simulink model "APP_MyApplication"  (R2018b)
settings: Solver=VariableStepDiscrete  StartTime=0.0  StopTime=10  RelTol=1e-3
PreLoadFcn:
  | if(exist('MBDS_ModelCallback', 'file')), MBDS_ModelCallback('PreLoad'); end;
PostLoadFcn:
  | if(exist('MBDS_ModelCallback', 'file')), MBDS_ModelCallback('PostLoad'); end;
InitFcn:
  | if(exist('MBDS_ModelCallback', 'file')), MBDS_ModelCallback('Init'); end;
StartFcn:
  | if(exist('MBDS_ModelCallback', 'file')), MBDS_ModelCallback('Start'); end;
StopFcn:
  | if(exist('MBDS_ModelCallback', 'file')), MBDS_ModelCallback('Stop'); end;
undefined symbols (not defined in the file): sigbuilder_block, Ts
libraries: KIBES_Signal x499, simulink x8
(part 2 of 10)

== system APP_MyApplication/Model/APP_MyApplication_/D-CAN(1) ==
  note: 18 01 01 F1
  Add : Sum  InitFcn=|  OutDataTypeStr=Inherit: Inherit via back propagation  SaturateOnIntegerOverflow=on
      | if(exist('MBDS_BlockCallback', 'file'))
      |    MBDS_BlockCallback('Update', gcb);  
      | end
      settings: AttributesFormatString=Saturate: %<SaturateOnIntegerOverflow>
  Constant1 : Constant  InitFcn=|  Value=0  OutDataTypeStr=boolean
      | if(exist('MBDS_BlockCallback', 'file'))
      |    MBDS_BlockCallback('Update', gcb);  
      | end
  Constant2 : Constant  InitFcn=|  OutDataTypeStr=boolean
      | if(exist('MBDS_BlockCallback', 'file'))
      |    MBDS_BlockCallback('Update', gcb);  
      | end
  Constant3 : Constant  InitFcn=|  Value=2  OutDataTypeStr=uint8
      | if(exist('MBDS_BlockCallback', 'file'))
      |    MBDS_BlockCallback('Update', gcb);  
      | end
  Constant4 : Constant  InitFcn=|  Value=3  OutDataTypeStr=uint8
      | if(exist('MBDS_BlockCallback', 'file'))
      |    MBDS_BlockCallback('Update', gcb);  
      | end
  Constant5 : Constant  InitFcn=|  Value=4  OutDataTypeStr=uint8
      | if(exist('MBDS_BlockCallback', 'file'))
      |    MBDS_BlockCallback('Update', gcb);  
      | end
  Constant6 : Constant  InitFcn=|  Value=1234  OutDataTypeStr=uint32
      | if(exist('MBDS_BlockCallback', 'file'))
      |    MBDS_BlockCallback('Update', gcb);  
      | end
  Constant7 : Constant  InitFcn=|  OutDataTypeStr=boolean
      | if(exist('MBDS_BlockCallback', 'file'))
      |    MBDS_BlockCallback('Update', gcb);  
      | end
  Constant9 : Constant  InitFcn=|  OutDataTypeStr=uint32
      | if(exist('MBDS_BlockCallback', 'file'))
      |    MBDS_BlockCallback('Update', gcb);  
      | end
  Data Type Conversion : DataTypeConversion  InitFcn=|  SaturateOnIntegerOverflow=on
      | try
      |    MBDS_BlockCallback('Update', gcb);
      | end
      settings: AttributesFormatString=Saturate: %<SaturateOnIntegerOverflow>
  NOT : Subsystem  InitFcn=|  mask(NOT){MBDS_LibraryBlock=on, BitwiseMode=off, Inputs=1, UseBitMask=off, BitMask='A1', OutDataTypeStr=Inherit: Inherit via back propagation, MBDS_BlockVersion=07.21.05}
      | if(exist('MBDS_BlockCallback', 'file'))
      |    MBDS_BlockCallback('Update', gcb);
      | end
      mask prompts: MBDS_LibraryBlock "MBDS library block"; BitwiseMode "Use 'bitwise' mode"; Inputs "Number of input ports:"; UseBitMask "Use bit mask"; BitMask "Bit mask:"; OutDataTypeStr "Output data type:"; MBDS_BlockVersion "Version:"
      mask help: Logical or bitwise NOT operator. The input value is inverted. In bitwise mode all bits of the input signal are inverted.
      mask init: same as APP_MyApplication/Model/APP_MyApplication_/OR
      mask Help: eval(['open([workdir(''library_dir:''),''\Blockset\help\'',get_param(gcb,''MaskType''),''.html''])'])
      mask Callback BitwiseMode:
      | if(exist('MBDS_BlockCallback', 'file'))
      |    MBDS_BlockCallback('BitwiseMode', gcb);
      | end
      mask TypeOptions OutDataTypeStr: Inherit: Inherit via back propagation | int8 | uint8 | int16 | uint16 | int32 | uint32 | boolean
      mask Callback OutDataTypeStr:
      | % Adopt Value
      | if(exist('MBDS_BlockCallback', 'file'))
      |    MBDS_BlockCallback('OutDataTypeStr', gcb);
      | end
      mask DialogControl ParameterTabVar0 Prompt: Main
      mask DialogControl ParameterTabVar01 Prompt: Signal Attributes
      mask DialogControl ParameterTabVar012 Prompt: Version
      mask Display:
      | % Show icon or block text
      | disp('NOT')
  in_DCAN.TX_Gen.DGenTx_4.MessageState : KIBES_Signal/KIBES_Signal  MBDS_LibraryBlock=on  DatabaseKey=271  SignalName=DCAN.TX_Gen.DGenTx_4.MessageState  SymbolName=DCAN_TX_Gen_DGenTx_4_MessageState_000271  DataType=uint16  Init=0  Slope=1  Bias=0  DataSize=1  fpDataType=uint16  BlockIOType=Inport  DeviceType=0
  in_DCAN.TX_Gen.DGenTx_4.Val1 : KIBES_Signal/KIBES_Signal  MBDS_LibraryBlock=on  DatabaseKey=272  SignalName=DCAN.TX_Gen.DGenTx_4.Val1  SymbolName=DCAN_TX_Gen_DGenTx_4_Val1_000272  DataType=uint32  Init=0  Slope=1  Bias=0  DataSize=1  fpDataType=uint32  BlockIOType=Inport  DeviceType=0
  in_IN_DCAN.RX_Gen.Test1.MessageState : KIBES_Signal/KIBES_Signal  MBDS_LibraryBlock=on  DatabaseKey=10  SignalName=IN_DCAN.RX_Gen.Test1.MessageState  SymbolName=IN_DCAN_RX_Gen_Test1_MessageState_000010  DataType=uint16  Init=0  Slope=1  Bias=0  DataSize=1  fpDataType=uint16  BlockIOType=Inport  DeviceType=0
  in_IN_DCAN.RX_Gen.Test1.Val1 : KIBES_Signal/KIBES_Signal  MBDS_LibraryBlock=on  DatabaseKey=11  SignalName=IN_DCAN.RX_Gen.Test1.Val1  SymbolName=IN_DCAN_RX_Gen_Test1_Val1_000011  DataType=uint8  Init=0  Slope=1  Bias=0  DataSize=1  fpDataType=uint8  BlockIOType=Inport  DeviceType=0
  in_IN_DCAN.TX_Gen.GenericTxMessage.MessageState : KIBES_Signal/KIBES_Signal  MBDS_LibraryBlock=on  DatabaseKey=3  SignalName=IN_DCAN.TX_Gen.GenericTxMessage.MessageState  SymbolName=IN_DCAN_TX_Gen_GenericTxMessage_MessageState_000003  DataType=uint16  Init=0  Slope=1  Bias=0  DataSize=1  fpDataType=uint16  BlockIOType=Inport  DeviceType=0
  in_STIMD.GenTxCycleTime : KIBES_Signal/KIBES_Signal  MBDS_LibraryBlock=on  DatabaseKey=576  SignalName=STIMD.GenTxCycleTime  SymbolName=STIMD_GenTxCycleTime_000576  DataType=uint16  Init=100  Slope=1  Bias=0  DataSize=1  fpDataType=uint16  BlockIOType=Inport  DeviceType=2
  out_DCAN.TX_Gen.DGenTx_4.MessageEnable : KIBES_Signal/KIBES_Signal  MBDS_LibraryBlock=on  DatabaseKey=270  SignalName=DCAN.TX_Gen.DGenTx_4.MessageEnable  SymbolName=DCAN_TX_Gen_DGenTx_4_MessageEnable_000270  DataType=boolean  Init=0  Slope=1  Bias=0  DataSize=1  fpDataType=boolean  BlockIOType=Outport  DeviceType=0
  out_DCAN.TX_Gen.DGenTx_4.Val1 : KIBES_Signal/KIBES_Signal  MBDS_LibraryBlock=on  DatabaseKey=272  SignalName=DCAN.TX_Gen.DGenTx_4.Val1  SymbolName=DCAN_TX_Gen_DGenTx_4_Val1_000272  DataType=uint32  Init=0  Slope=1  Bias=0  DataSize=1  fpDataType=uint32  BlockIOType=Outport  DeviceType=0
  out_DCAN.TX_Gen.GenericTxMessage.CycleTime : KIBES_Signal/KIBES_Signal  MBDS_LibraryBlock=on  DatabaseKey=575  SignalName=DCAN.TX_Gen.GenericTxMessage.CycleTime  SymbolName=DCAN_TX_Gen_GenericTxMessage_CycleTime_000575  DataType=uint16  Init=0  Slope=1  Bias=0  DataSize=1  fpDataType=uint16  BlockIOType=Outport  DeviceType=0
  out_OUT_DCAN.RX_Gen.Test1.MessageEnable : KIBES_Signal/KIBES_Signal  MBDS_LibraryBlock=on  DatabaseKey=9  SignalName=OUT_DCAN.RX_Gen.Test1.MessageEnable  SymbolName=OUT_DCAN_RX_Gen_Test1_MessageEnable_000009  DataType=boolean  Init=0  Slope=1  Bias=0  DataSize=1  fpDataType=boolean  BlockIOType=Outport  DeviceType=0
  out_OUT_DCAN.TX_Gen.GenericTxMessage.MessageEnable : KIBES_Signal/KIBES_Signal  MBDS_LibraryBlock=on  DatabaseKey=2  SignalName=OUT_DCAN.TX_Gen.GenericTxMessage.MessageEnable  SymbolName=OUT_DCAN_TX_Gen_GenericTxMessage_MessageEnable_000002  DataType=boolean  Init=0  Slope=1  Bias=0  DataSize=1  fpDataType=boolean  BlockIOType=Outport  DeviceType=0
  out_OUT_DCAN.TX_Gen.GenericTxMessage.Val1 : KIBES_Signal/KIBES_Signal  MBDS_LibraryBlock=on  DatabaseKey=4  SignalName=OUT_DCAN.TX_Gen.GenericTxMessage.Val1  SymbolName=OUT_DCAN_TX_Gen_GenericTxMessage_Val1_000004  DataType=uint8  Init=0  Slope=1  Bias=0  DataSize=1  fpDataType=uint8  BlockIOType=Outport  DeviceType=0
  out_OUT_DCAN.TX_Gen.GenericTxMessage.Val2 : KIBES_Signal/KIBES_Signal  MBDS_LibraryBlock=on  DatabaseKey=5  SignalName=OUT_DCAN.TX_Gen.GenericTxMessage.Val2  SymbolName=OUT_DCAN_TX_Gen_GenericTxMessage_Val2_000005  DataType=uint8  Init=0  Slope=1  Bias=0  DataSize=1  fpDataType=uint8  BlockIOType=Outport  DeviceType=0
  out_OUT_DCAN.TX_Gen.GenericTxMessage.Val3 : KIBES_Signal/KIBES_Signal  MBDS_LibraryBlock=on  DatabaseKey=6  SignalName=OUT_DCAN.TX_Gen.GenericTxMessage.Val3  SymbolName=OUT_DCAN_TX_Gen_GenericTxMessage_Val3_000006  DataType=uint8  Init=0  Slope=1  Bias=0  DataSize=1  fpDataType=uint8  BlockIOType=Outport  DeviceType=0
  out_OUT_DCAN.TX_Gen.GenericTxMessage.Val4 : KIBES_Signal/KIBES_Signal  MBDS_LibraryBlock=on  DatabaseKey=7  SignalName=OUT_DCAN.TX_Gen.GenericTxMessage.Val4  SymbolName=OUT_DCAN_TX_Gen_GenericTxMessage_Val4_000007  DataType=uint8  Init=0  Slope=1  Bias=0  DataSize=1  fpDataType=uint8  BlockIOType=Outport  DeviceType=0
  out_OUT_DCAN.TX_Gen.GenericTxMessage.Val5 : KIBES_Signal/KIBES_Signal  MBDS_LibraryBlock=on  DatabaseKey=8  SignalName=OUT_DCAN.TX_Gen.GenericTxMessage.Val5  SymbolName=OUT_DCAN_TX_Gen_GenericTxMessage_Val5_000008  DataType=uint32  Init=0  Slope=1  Bias=0  DataSize=1  fpDataType=uint32  BlockIOType=Outport  DeviceType=0
  wires:
  Add/1 -> out_DCAN.TX_Gen.DGenTx_4.Val1/1
  in_DCAN.TX_Gen.DGenTx_4.Val1/1 -> Add/1
  Constant9/1 -> Add/2
  Constant6/1 -> out_OUT_DCAN.TX_Gen.GenericTxMessage.Val5/1
  in_STIMD.GenTxCycleTime/1 -> out_DCAN.TX_Gen.GenericTxMessage.CycleTime/1
  Data Type Conversion/1 -> NOT/1(u1)
  Constant5/1 -> out_OUT_DCAN.TX_Gen.GenericTxMessage.Val4/1
  Constant3/1 -> out_OUT_DCAN.TX_Gen.GenericTxMessage.Val2/1
  Constant7/1 -> out_OUT_DCAN.RX_Gen.Test1.MessageEnable/1
  in_IN_DCAN.RX_Gen.Test1.MessageState/1 -> Data Type Conversion/1
  Constant4/1 -> out_OUT_DCAN.TX_Gen.GenericTxMessage.Val3/1
  in_IN_DCAN.RX_Gen.Test1.Val1/1 -> out_OUT_DCAN.TX_Gen.GenericTxMessage.Val1/1
  NOT/1(y) -> out_OUT_DCAN.TX_Gen.GenericTxMessage.MessageEnable/1
  Constant2/1 -> out_DCAN.TX_Gen.DGenTx_4.MessageEnable/1

== system APP_MyApplication/Model/APP_MyApplication_/DM13 ==
  Constant1 : Constant  InitFcn=|  Value=0  OutDataTypeStr=boolean
      | if(exist('MBDS_BlockCallback', 'file'))
      |    MBDS_BlockCallback('Update', gcb);  
      | end
  Data Type Conversion : DataTypeConversion  InitFcn=|  SaturateOnIntegerOverflow=on
      | try
      |    MBDS_BlockCallback('Update', gcb);
      | end
      settings: AttributesFormatString=Saturate: %<SaturateOnIntegerOverflow>
  OR1 : Subsystem  InitFcn=|  mask(OR){MBDS_LibraryBlock=on, BitwiseMode=off, Inputs=2, UseBitMask=off, BitMask='A1', OutDataTypeStr=Inherit: Inherit via back propagation, MBDS_BlockVersion=07.21.05}
      | if(exist('MBDS_BlockCallback', 'file'))
      |    MBDS_BlockCallback('Update', gcb);
      | end
      mask prompts: MBDS_LibraryBlock "MBDS library block"; BitwiseMode "Use 'bitwise' mode"; Inputs "Number of input ports:"; UseBitMask "Use bit mask"; BitMask "Bit mask:"; OutDataTypeStr "Output data type:"; MBDS_BlockVersion "Version:"
      mask help: Logical or bitwise OR operator. For multiple inputs, operators are applied across the inputs. For a single input, operators are applied across the input vector. In bitwise mode a bit mask can be applied onto single input signals.
      mask init: same as APP_MyApplication/Model/APP_MyApplication_/OR
      mask Help: eval(['open([workdir(''library_dir:''),''\Blockset\help\'',get_param(gcb,''MaskType''),''.html''])'])
      mask Callback BitwiseMode:
      | if(exist('MBDS_BlockCallback', 'file'))
      |    MBDS_BlockCallback('BitwiseMode', gcb);
      | end
      mask Callback Inputs:
      | if(exist('MBDS_BlockCallback', 'file'))
      |    MBDS_BlockCallback('Inputs', gcb);
      | end
      mask Callback UseBitMask:
      | if(exist('MBDS_BlockCallback', 'file'))
      |    MBDS_BlockCallback('UseBitMask', gcb);
      | end
      mask Callback BitMask:
      | if(exist('MBDS_BlockCallback', 'file'))
      |    MBDS_BlockCallback('BitMask', gcb);
      | end
      mask TypeOptions OutDataTypeStr: Inherit: Inherit via back propagation | int8 | uint8 | int16 | uint16 | int32 | uint32 | boolean
      mask Callback OutDataTypeStr:
      | % Adopt Value
      | if(exist('MBDS_BlockCallback', 'file'))
      |    MBDS_BlockCallback('OutDataTypeStr', gcb);
      | end
      mask DialogControl ParameterTabVar0 Prompt: Main
      mask DialogControl ParameterTabVar01 Prompt: Signal Attributes
      mask DialogControl ParameterTabVar012 Prompt: Version
      mask Display:
      | % Show icon or block text
      | if(UseBitMask)
      |    if(isnumeric(BitMask))
      |       BitMaskString = ['0x',dec2hex(floor(BitMask))];
      |    elseif(ischar(BitMask))
      |       BitMaskString = ['0x',upper(BitMask)];
      |    else
      |       BitMaskString = '???';
      |    end
      |    disp(sprintf(['OR\n', BitMaskString]))
      | else
      |    disp('OR')
      | end
  in_DCAN.BusOffState : KIBES_Signal/KIBES_Signal  MBDS_LibraryBlock=on  DatabaseKey=639  SignalName=DCAN.BusOffState  SymbolName=DCAN_BusOffState_000639  DataType=boolean  Init=0  Slope=1  Bias=0  DataSize=1  fpDataType=boolean  BlockIOType=Inport  DeviceType=0
  in_DCAN.GenericDM13RXMessage.CurrentDataLink : KIBES_Signal/KIBES_Signal  MBDS_LibraryBlock=on  DatabaseKey=366  SignalName=DCAN.GenericDM13RXMessage.CurrentDataLink  SymbolName=DCAN_GenericDM13RXMessage_CurrentDataLink_000366  DataType=boolean  Init=0  Slope=1  Bias=0  DataSize=1  fpDataType=boolean  BlockIOType=Inport  DeviceType=0
  in_DCAN.GenericDM13RXMessage.CurrentDataLink_DIAG : KIBES_Signal/KIBES_Signal  MBDS_LibraryBlock=on  DatabaseKey=365  SignalName=DCAN.GenericDM13RXMessage.CurrentDataLink_DIAG  SymbolName=DCAN_GenericDM13RXMessage_CurrentDataLink_DIAG_000365  DataType=uint16  Init=1  Slope=1  Bias=0  DataSize=1  fpDataType=uint16  BlockIOType=Inport  DeviceType=0
  in_DCAN.GenericDM13RXMessage.DataChangeIndicator : KIBES_Signal/KIBES_Signal  MBDS_LibraryBlock=on  DatabaseKey=364  SignalName=DCAN.GenericDM13RXMessage.DataChangeIndicator  SymbolName=DCAN_GenericDM13RXMessage_DataChangeIndicator_000364  DataType=boolean  Init=0  Slope=1  Bias=0  DataSize=1  fpDataType=boolean  BlockIOType=Inport  DeviceType=0
  in_DCAN.GenericDM13RXMessage.DeviceState : KIBES_Signal/KIBES_Signal  MBDS_LibraryBlock=on  DatabaseKey=362  SignalName=DCAN.GenericDM13RXMessage.DeviceState  SymbolName=DCAN_GenericDM13RXMessage_DeviceState_000362  DataType=uint16  Init=0  Slope=1  Bias=0  DataSize=1  fpDataType=uint16  BlockIOType=Inport  DeviceType=0
  in_DCAN.GenericDM13RXMessage.ISO9141 : KIBES_Signal/KIBES_Signal  MBDS_LibraryBlock=on  DatabaseKey=361  SignalName=DCAN.GenericDM13RXMessage.ISO9141  SymbolName=DCAN_GenericDM13RXMessage_ISO9141_000361  DataType=boolean  Init=0  Slope=1  Bias=0  DataSize=1  fpDataType=boolean  BlockIOType=Inport  DeviceType=0
  in_DCAN.GenericDM13RXMessage.ISO9141_DIAG : KIBES_Signal/KIBES_Signal  MBDS_LibraryBlock=on  DatabaseKey=360  SignalName=DCAN.GenericDM13RXMessage.ISO9141_DIAG  SymbolName=DCAN_GenericDM13RXMessage_ISO9141_DIAG_000360  DataType=uint16  Init=1  Slope=1  Bias=0  DataSize=1  fpDataType=uint16  BlockIOType=Inport  DeviceType=0
  in_DCAN.GenericDM13RXMessage.J1587 : KIBES_Signal/KIBES_Signal  MBDS_LibraryBlock=on  DatabaseKey=359  SignalName=DCAN.GenericDM13RXMessage.J1587  SymbolName=DCAN_GenericDM13RXMessage_J1587_000359  DataType=boolean  Init=0  Slope=1  Bias=0  DataSize=1  fpDataType=boolean  BlockIOType=Inport  DeviceType=0
  in_DCAN.GenericDM13RXMessage.J1587_DIAG : KIBES_Signal/KIBES_Signal  MBDS_LibraryBlock=on  DatabaseKey=358  SignalName=DCAN.GenericDM13RXMessage.J1587_DIAG  SymbolName=DCAN_GenericDM13RXMessage_J1587_DIAG_000358  DataType=uint16  Init=1  Slope=1  Bias=0  DataSize=1  fpDataType=uint16  BlockIOType=Inport  DeviceType=0
  in_DCAN.GenericDM13RXMessage.J1850 : KIBES_Signal/KIBES_Signal  MBDS_LibraryBlock=on  DatabaseKey=357  SignalName=DCAN.GenericDM13RXMessage.J1850  SymbolName=DCAN_GenericDM13RXMessage_J1850_000357  DataType=boolean  Init=0  Slope=1  Bias=0  DataSize=1  fpDataType=boolean  BlockIOType=Inport  DeviceType=0
  in_DCAN.GenericDM13RXMessage.J1850_DIAG : KIBES_Signal/KIBES_Signal  MBDS_LibraryBlock=on  DatabaseKey=356  SignalName=DCAN.GenericDM13RXMessage.J1850_DIAG  SymbolName=DCAN_GenericDM13RXMessage_J1850_DIAG_000356  DataType=uint16  Init=1  Slope=1  Bias=0  DataSize=1  fpDataType=uint16  BlockIOType=Inport  DeviceType=0
  in_DCAN.GenericDM13RXMessage.J1922 : KIBES_Signal/KIBES_Signal  MBDS_LibraryBlock=on  DatabaseKey=355  SignalName=DCAN.GenericDM13RXMessage.J1922  SymbolName=DCAN_GenericDM13RXMessage_J1922_000355  DataType=boolean  Init=0  Slope=1  Bias=0  DataSize=1  fpDataType=boolean  BlockIOType=Inport  DeviceType=0
  in_DCAN.GenericDM13RXMessage.J1922_DIAG : KIBES_Signal/KIBES_Signal  MBDS_LibraryBlock=on  DatabaseKey=354  SignalName=DCAN.GenericDM13RXMessage.J1922_DIAG  SymbolName=DCAN_GenericDM13RXMessage_J1922_DIAG_000354  DataType=uint16  Init=1  Slope=1  Bias=0  DataSize=1  fpDataType=uint16  BlockIOType=Inport  DeviceType=0
  in_DCAN.GenericDM13RXMessage.Network1 : KIBES_Signal/KIBES_Signal  MBDS_LibraryBlock=on  DatabaseKey=353  SignalName=DCAN.GenericDM13RXMessage.Network1  SymbolName=DCAN_GenericDM13RXMessage_Network1_000353  DataType=boolean  Init=0  Slope=1  Bias=0  DataSize=1  fpDataType=boolean  BlockIOType=Inport  DeviceType=0
  in_DCAN.GenericDM13RXMessage.Network1_DIAG : KIBES_Signal/KIBES_Signal  MBDS_LibraryBlock=on  DatabaseKey=352  SignalName=DCAN.GenericDM13RXMessage.Network1_DIAG  SymbolName=DCAN_GenericDM13RXMessage_Network1_DIAG_000352  DataType=uint16  Init=1  Slope=1  Bias=0  DataSize=1  fpDataType=uint16  BlockIOType=Inport  DeviceType=0
  in_DCAN.GenericDM13RXMessage.Network2 : KIBES_Signal/KIBES_Signal  MBDS_LibraryBlock=on  DatabaseKey=351  SignalName=DCAN.GenericDM13RXMessage.Network2  SymbolName=DCAN_GenericDM13RXMessage_Network2_000351  DataType=boolean  Init=0  Slope=1  Bias=0  DataSize=1  fpDataType=boolean  BlockIOType=Inport  DeviceType=0
  in_DCAN.GenericDM13RXMessage.Network2_DIAG : KIBES_Signal/KIBES_Signal  MBDS_LibraryBlock=on  DatabaseKey=350  SignalName=DCAN.GenericDM13RXMessage.Network2_DIAG  SymbolName=DCAN_GenericDM13RXMessage_Network2_DIAG_000350  DataType=uint16  Init=1  Slope=1  Bias=0  DataSize=1  fpDataType=uint16  BlockIOType=Inport  DeviceType=0
  in_DCAN.GenericDM13RXMessage.Network3 : KIBES_Signal/KIBES_Signal  MBDS_LibraryBlock=on  DatabaseKey=349  SignalName=DCAN.GenericDM13RXMessage.Network3  SymbolName=DCAN_GenericDM13RXMessage_Network3_000349  DataType=boolean  Init=0  Slope=1  Bias=0  DataSize=1  fpDataType=boolean  BlockIOType=Inport  DeviceType=0
  in_DCAN.GenericDM13RXMessage.Network3_DIAG : KIBES_Signal/KIBES_Signal  MBDS_LibraryBlock=on  DatabaseKey=348  SignalName=DCAN.GenericDM13RXMessage.Network3_DIAG  SymbolName=DCAN_GenericDM13RXMessage_Network3_DIAG_000348  DataType=uint16  Init=1  Slope=1  Bias=0  DataSize=1  fpDataType=uint16  BlockIOType=Inport  DeviceType=0
  in_DCAN.GenericDM13RXMessage.OtherManufacturer : KIBES_Signal/KIBES_Signal  MBDS_LibraryBlock=on  DatabaseKey=347  SignalName=DCAN.GenericDM13RXMessage.OtherManufacturer  SymbolName=DCAN_GenericDM13RXMessage_OtherManufacturer_000347  DataType=boolean  Init=0  Slope=1  Bias=0  DataSize=1  fpDataType=boolean  BlockIOType=Inport  DeviceType=0
  in_DCAN.GenericDM13RXMessage.OtherManufacturer_DIAG : KIBES_Signal/KIBES_Signal  MBDS_LibraryBlock=on  DatabaseKey=346  SignalName=DCAN.GenericDM13RXMessage.OtherManufacturer_DIAG  SymbolName=DCAN_GenericDM13RXMessage_OtherManufacturer_DIAG_000346  DataType=uint16  Init=1  Slope=1  Bias=0  DataSize=1  fpDataType=uint16  BlockIOType=Inport  DeviceType=0
  in_STIMD.DM13_enable : KIBES_Signal/KIBES_Signal  MBDS_LibraryBlock=on  DatabaseKey=367  SignalName=STIMD.DM13_enable  SymbolName=STIMD_DM13_enable_000367  DataType=boolean  Init=0  Slope=1  Bias=0  DataSize=1  fpDataType=boolean  BlockIOType=Inport  DeviceType=2
  out_DCAN.GenericDM13RXMessage.DeviceEnable : KIBES_Signal/KIBES_Signal  MBDS_LibraryBlock=on  DatabaseKey=363  SignalName=DCAN.GenericDM13RXMessage.DeviceEnable  SymbolName=DCAN_GenericDM13RXMessage_DeviceEnable_000363  DataType=boolean  Init=0  Slope=1  Bias=0  DataSize=1  fpDataType=boolean  BlockIOType=Outport  DeviceType=0
  out_PCAN.TX_GEN.PGenTX_3.MessageEnable : KIBES_Signal/KIBES_Signal  MBDS_LibraryBlock=on  DatabaseKey=640  SignalName=PCAN.TX_GEN.PGenTX_3.MessageEnable  SymbolName=PCAN_TX_GEN_PGenTX_3_MessageEnable_000640  DataType=boolean  Init=0  Slope=1  Bias=0  DataSize=1  fpDataType=boolean  BlockIOType=Outport  DeviceType=0
  out_PCAN.TX_GEN.PGenTX_3.ui_Val_02 : KIBES_Signal/KIBES_Signal  MBDS_LibraryBlock=on  DatabaseKey=642  SignalName=PCAN.TX_GEN.PGenTX_3.ui_Val_02  SymbolName=PCAN_TX_GEN_PGenTX_3_ui_Val_02_000642  DataType=uint16  Init=0  Slope=1  Bias=0  DataSize=1  fpDataType=uint16  BlockIOType=Outport  DeviceType=0
  out_PCAN.TX_GEN.PGenTX_3.usi_Val_01 : KIBES_Signal/KIBES_Signal  MBDS_LibraryBlock=on  DatabaseKey=641  SignalName=PCAN.TX_GEN.PGenTX_3.usi_Val_01  SymbolName=PCAN_TX_GEN_PGenTX_3_usi_Val_01_000641  DataType=uint8  Init=0  Slope=1  Bias=0  DataSize=1  fpDataType=uint8  BlockIOType=Outport  DeviceType=0
  wires:
  OR1/1(y) -> out_DCAN.GenericDM13RXMessage.DeviceEnable/1, out_PCAN.TX_GEN.PGenTX_3.MessageEnable/1
  Constant1/1 -> OR1/2(u2)
  in_STIMD.DM13_enable/1 -> OR1/1(u1)
  in_DCAN.GenericDM13RXMessage.DeviceState/1 -> out_PCAN.TX_GEN.PGenTX_3.ui_Val_02/1
  Data Type Conversion/1 -> out_PCAN.TX_GEN.PGenTX_3.usi_Val_01/1
  in_DCAN.BusOffState/1 -> Data Type Conversion/1

== system APP_MyApplication/Model/APP_MyApplication_/DM1TX ==
  note: DM1TX
  in_DCAN.GenericDM1TxMessage.DeviceState : KIBES_Signal/KIBES_Signal  MBDS_LibraryBlock=on  DatabaseKey=202  SignalName=DCAN.GenericDM1TxMessage.DeviceState  SymbolName=DCAN_GenericDM1TxMessage_DeviceState_000202  DataType=uint16  Init=0  Slope=1  Bias=0  DataSize=1  fpDataType=uint16  BlockIOType=Inport  DeviceType=0
  in_FMSCAN.GenericDM1TxMessage.DeviceState : KIBES_Signal/KIBES_Signal  MBDS_LibraryBlock=on  DatabaseKey=340  SignalName=FMSCAN.GenericDM1TxMessage.DeviceState  SymbolName=FMSCAN_GenericDM1TxMessage_DeviceState_000340  DataType=uint16  Init=0  Slope=1  Bias=0  DataSize=1  fpDataType=uint16  BlockIOType=Inport  DeviceType=0
  in_PCAN.GenericDM1TxMessage.DeviceState : KIBES_Signal/KIBES_Signal  MBDS_LibraryBlock=on  DatabaseKey=338  SignalName=PCAN.GenericDM1TxMessage.DeviceState  SymbolName=PCAN_GenericDM1TxMessage_DeviceState_000338  DataType=uint16  Init=0  Slope=1  Bias=0  DataSize=1  fpDataType=uint16  BlockIOType=Inport  DeviceType=0
  in_STIMD.D_DM1TX : KIBES_Signal/KIBES_Signal  MBDS_LibraryBlock=on  DatabaseKey=636  SignalName=STIMD.D_DM1TX  SymbolName=STIMD_D_DM1TX_000636  DataType=boolean  Init=0  Slope=1  Bias=0  DataSize=1  fpDataType=boolean  BlockIOType=Inport  DeviceType=2
  in_STIMD.F_DM1TX : KIBES_Signal/KIBES_Signal  MBDS_LibraryBlock=on  DatabaseKey=637  SignalName=STIMD.F_DM1TX  SymbolName=STIMD_F_DM1TX_000637  DataType=boolean  Init=0  Slope=1  Bias=0  DataSize=1  fpDataType=boolean  BlockIOType=Inport  DeviceType=2
  in_STIMD.P_DM1TX : KIBES_Signal/KIBES_Signal  MBDS_LibraryBlock=on  DatabaseKey=635  SignalName=STIMD.P_DM1TX  SymbolName=STIMD_P_DM1TX_000635  DataType=boolean  Init=0  Slope=1  Bias=0  DataSize=1  fpDataType=boolean  BlockIOType=Inport  DeviceType=2
  out_DCAN.GenericDM1TxMessage.DeviceEnable : KIBES_Signal/KIBES_Signal  MBDS_LibraryBlock=on  DatabaseKey=201  SignalName=DCAN.GenericDM1TxMessage.DeviceEnable  SymbolName=DCAN_GenericDM1TxMessage_DeviceEnable_000201  DataType=boolean  Init=0  Slope=1  Bias=0  DataSize=1  fpDataType=boolean  BlockIOType=Outport  DeviceType=0
  out_FMSCAN.GenericDM1TxMessage.DeviceEnable : KIBES_Signal/KIBES_Signal  MBDS_LibraryBlock=on  DatabaseKey=341  SignalName=FMSCAN.GenericDM1TxMessage.DeviceEnable  SymbolName=FMSCAN_GenericDM1TxMessage_DeviceEnable_000341  DataType=boolean  Init=0  Slope=1  Bias=0  DataSize=1  fpDataType=boolean  BlockIOType=Outport  DeviceType=0
  out_PCAN.GenericDM1TxMessage.DeviceEnable : KIBES_Signal/KIBES_Signal  MBDS_LibraryBlock=on  DatabaseKey=339  SignalName=PCAN.GenericDM1TxMessage.DeviceEnable  SymbolName=PCAN_GenericDM1TxMessage_DeviceEnable_000339  DataType=boolean  Init=0  Slope=1  Bias=0  DataSize=1  fpDataType=boolean  BlockIOType=Outport  DeviceType=0
  wires:
  in_STIMD.D_DM1TX/1 -> out_DCAN.GenericDM1TxMessage.DeviceEnable/1
  in_STIMD.P_DM1TX/1 -> out_PCAN.GenericDM1TxMessage.DeviceEnable/1
  in_STIMD.F_DM1TX/1 -> out_FMSCAN.GenericDM1TxMessage.DeviceEnable/1

== system APP_MyApplication/Model/APP_MyApplication_/DM2_3_11 ==
  Constant1 : Constant  InitFcn=|  OutDataTypeStr=boolean
      | if(exist('MBDS_BlockCallback', 'file'))
      |    MBDS_BlockCallback('Update', gcb);  
      | end
  Constant2 : Constant  InitFcn=|  OutDataTypeStr=boolean
      | if(exist('MBDS_BlockCallback', 'file'))
      |    MBDS_BlockCallback('Update', gcb);  
      | end
  Constant3 : Constant  InitFcn=|  OutDataTypeStr=boolean
      | if(exist('MBDS_BlockCallback', 'file'))
      |    MBDS_BlockCallback('Update', gcb);  
      | end
  OR1 : Subsystem  InitFcn=|  mask(OR){MBDS_LibraryBlock=on, BitwiseMode=off, Inputs=2, UseBitMask=off, BitMask='A1', OutDataTypeStr=Inherit: Inherit via back propagation, MBDS_BlockVersion=07.21.05}
      | if(exist('MBDS_BlockCallback', 'file'))
      |    MBDS_BlockCallback('Update', gcb);
      | end
      mask prompts: MBDS_LibraryBlock "MBDS library block"; BitwiseMode "Use 'bitwise' mode"; Inputs "Number of input ports:"; UseBitMask "Use bit mask"; BitMask "Bit mask:"; OutDataTypeStr "Output data type:"; MBDS_BlockVersion "Version:"
      mask help: Logical or bitwise OR operator. For multiple inputs, operators are applied across the inputs. For a single input, operators are applied across the input vector. In bitwise mode a bit mask can be applied onto single input signals.
      mask init: same as APP_MyApplication/Model/APP_MyApplication_/OR
      mask Help: eval(['open([workdir(''library_dir:''),''\Blockset\help\'',get_param(gcb,''MaskType''),''.html''])'])
      mask Callback BitwiseMode:
      | if(exist('MBDS_BlockCallback', 'file'))
      |    MBDS_BlockCallback('BitwiseMode', gcb);
      | end
      mask Callback Inputs:
      | if(exist('MBDS_BlockCallback', 'file'))
      |    MBDS_BlockCallback('Inputs', gcb);
      | end
      mask Callback UseBitMask:
      | if(exist('MBDS_BlockCallback', 'file'))
      |    MBDS_BlockCallback('UseBitMask', gcb);
      | end
      mask Callback BitMask:
      | if(exist('MBDS_BlockCallback', 'file'))
      |    MBDS_BlockCallback('BitMask', gcb);
      | end
      mask TypeOptions OutDataTypeStr: Inherit: Inherit via back propagation | int8 | uint8 | int16 | uint16 | int32 | uint32 | boolean
      mask Callback OutDataTypeStr:
      | % Adopt Value
      | if(exist('MBDS_BlockCallback', 'file'))
      |    MBDS_BlockCallback('OutDataTypeStr', gcb);
      | end
      mask DialogControl ParameterTabVar0 Prompt: Main
      mask DialogControl ParameterTabVar01 Prompt: Signal Attributes
      mask DialogControl ParameterTabVar012 Prompt: Version
      mask Display:
      | % Show icon or block text
      | if(UseBitMask)
      |    if(isnumeric(BitMask))
      |       BitMaskString = ['0x',dec2hex(floor(BitMask))];
      |    elseif(ischar(BitMask))
      |       BitMaskString = ['0x',upper(BitMask)];
      |    else
      |       BitMaskString = '???';
      |    end
      |    disp(sprintf(['OR\n', BitMaskString]))
      | else
      |    disp('OR')
      | end
  OR2 : Subsystem  InitFcn=|  mask(OR){MBDS_LibraryBlock=on, BitwiseMode=off, Inputs=2, UseBitMask=off, BitMask='A1', OutDataTypeStr=Inherit: Inherit via back propagation, MBDS_BlockVersion=07.21.05}
      | if(exist('MBDS_BlockCallback', 'file'))
      |    MBDS_BlockCallback('Update', gcb);
      | end
      mask prompts: MBDS_LibraryBlock "MBDS library block"; BitwiseMode "Use 'bitwise' mode"; Inputs "Number of input ports:"; UseBitMask "Use bit mask"; BitMask "Bit mask:"; OutDataTypeStr "Output data type:"; MBDS_BlockVersion "Version:"
      mask help: Logical or bitwise OR operator. For multiple inputs, operators are applied across the inputs. For a single input, operators are applied across the input vector. In bitwise mode a bit mask can be applied onto single input signals.
      mask init: same as APP_MyApplication/Model/APP_MyApplication_/OR
      mask Help: eval(['open([workdir(''library_dir:''),''\Blockset\help\'',get_param(gcb,''MaskType''),''.html''])'])
      mask Callback BitwiseMode:
      | if(exist('MBDS_BlockCallback', 'file'))
      |    MBDS_BlockCallback('BitwiseMode', gcb);
      | end
      mask Callback Inputs:
      | if(exist('MBDS_BlockCallback', 'file'))
      |    MBDS_BlockCallback('Inputs', gcb);
      | end
      mask Callback UseBitMask:
      | if(exist('MBDS_BlockCallback', 'file'))
      |    MBDS_BlockCallback('UseBitMask', gcb);
      | end
      mask Callback BitMask:
      | if(exist('MBDS_BlockCallback', 'file'))
      |    MBDS_BlockCallback('BitMask', gcb);
      | end
      mask TypeOptions OutDataTypeStr: Inherit: Inherit via back propagation | int8 | uint8 | int16 | uint16 | int32 | uint32 | boolean
      mask Callback OutDataTypeStr:
      | % Adopt Value
      | if(exist('MBDS_BlockCallback', 'file'))
      |    MBDS_BlockCallback('OutDataTypeStr', gcb);
      | end
      mask DialogControl ParameterTabVar0 Prompt: Main
      mask DialogControl ParameterTabVar01 Prompt: Signal Attributes
      mask DialogControl ParameterTabVar012 Prompt: Version
      mask Display:
      | % Show icon or block text
      | if(UseBitMask)
      |    if(isnumeric(BitMask))
      |       BitMaskString = ['0x',dec2hex(floor(BitMask))];
      |    elseif(ischar(BitMask))
      |       BitMaskString = ['0x',upper(BitMask)];
      |    else
      |       BitMaskString = '???';
      |    end
      |    disp(sprintf(['OR\n', BitMaskString]))
      | else
      |    disp('OR')
      | end
  OR3 : Subsystem  InitFcn=|  mask(OR){MBDS_LibraryBlock=on, BitwiseMode=off, Inputs=2, UseBitMask=off, BitMask='A1', OutDataTypeStr=Inherit: Inherit via back propagation, MBDS_BlockVersion=07.21.05}
      | if(exist('MBDS_BlockCallback', 'file'))
      |    MBDS_BlockCallback('Update', gcb);
      | end
      mask prompts: MBDS_LibraryBlock "MBDS library block"; BitwiseMode "Use 'bitwise' mode"; Inputs "Number of input ports:"; UseBitMask "Use bit mask"; BitMask "Bit mask:"; OutDataTypeStr "Output data type:"; MBDS_BlockVersion "Version:"
      mask help: Logical or bitwise OR operator. For multiple inputs, operators are applied across the inputs. For a single input, operators are applied across the input vector. In bitwise mode a bit mask can be applied onto single input signals.
      mask init: same as APP_MyApplication/Model/APP_MyApplication_/OR
      mask Help: eval(['open([workdir(''library_dir:''),''\Blockset\help\'',get_param(gcb,''MaskType''),''.html''])'])
      mask Callback BitwiseMode:
      | if(exist('MBDS_BlockCallback', 'file'))
      |    MBDS_BlockCallback('BitwiseMode', gcb);
      | end
      mask Callback Inputs:
      | if(exist('MBDS_BlockCallback', 'file'))
      |    MBDS_BlockCallback('Inputs', gcb);
      | end
      mask Callback UseBitMask:
      | if(exist('MBDS_BlockCallback', 'file'))
      |    MBDS_BlockCallback('UseBitMask', gcb);
      | end
      mask Callback BitMask:
      | if(exist('MBDS_BlockCallback', 'file'))
      |    MBDS_BlockCallback('BitMask', gcb);
      | end
      mask TypeOptions OutDataTypeStr: Inherit: Inherit via back propagation | int8 | uint8 | int16 | uint16 | int32 | uint32 | boolean
      mask Callback OutDataTypeStr:
      | % Adopt Value
      | if(exist('MBDS_BlockCallback', 'file'))
      |    MBDS_BlockCallback('OutDataTypeStr', gcb);
      | end
      mask DialogControl ParameterTabVar0 Prompt: Main
      mask DialogControl ParameterTabVar01 Prompt: Signal Attributes
      mask DialogControl ParameterTabVar012 Prompt: Version
      mask Display:
      | % Show icon or block text
      | if(UseBitMask)
      |    if(isnumeric(BitMask))
      |       BitMaskString = ['0x',dec2hex(floor(BitMask))];
      |    elseif(ischar(BitMask))
      |       BitMaskString = ['0x',upper(BitMask)];
      |    else
      |       BitMaskString = '???';
      |    end
      |    disp(sprintf(['OR\n', BitMaskString]))
      | else
      |    disp('OR')
      | end
  in_DCAN.GenericDM11RXMessage.DeviceState : KIBES_Signal/KIBES_Signal  MBDS_LibraryBlock=on  DatabaseKey=396  SignalName=DCAN.GenericDM11RXMessage.DeviceState  SymbolName=DCAN_GenericDM11RXMessage_DeviceState_000396  DataType=uint16  Init=0  Slope=1  Bias=0  DataSize=1  fpDataType=uint16  BlockIOType=Inport  DeviceType=0
  in_DCAN.GenericDM2TxMessage.Device_State : KIBES_Signal/KIBES_Signal  MBDS_LibraryBlock=on  DatabaseKey=392  SignalName=DCAN.GenericDM2TxMessage.Device_State  SymbolName=DCAN_GenericDM2TxMessage_Device_State_000392  DataType=uint16  Init=0  Slope=1  Bias=0  DataSize=1  fpDataType=uint16  BlockIOType=Inport  DeviceType=0
  in_DCAN.GenericDM3RxMessage.Device_State : KIBES_Signal/KIBES_Signal  MBDS_LibraryBlock=on  DatabaseKey=394  SignalName=DCAN.GenericDM3RxMessage.Device_State  SymbolName=DCAN_GenericDM3RxMessage_Device_State_000394  DataType=uint16  Init=0  Slope=1  Bias=0  DataSize=1  fpDataType=uint16  BlockIOType=Inport  DeviceType=0
  in_STIMD.DM11_enable : KIBES_Signal/KIBES_Signal  MBDS_LibraryBlock=on  DatabaseKey=398  SignalName=STIMD.DM11_enable  SymbolName=STIMD_DM11_enable_000398  DataType=boolean  Init=0  Slope=1  Bias=0  DataSize=1  fpDataType=boolean  BlockIOType=Inport  DeviceType=2
  in_STIMD.DM2_enable : KIBES_Signal/KIBES_Signal  MBDS_LibraryBlock=on  DatabaseKey=399  SignalName=STIMD.DM2_enable  SymbolName=STIMD_DM2_enable_000399  DataType=boolean  Init=0  Slope=1  Bias=0  DataSize=1  fpDataType=boolean  BlockIOType=Inport  DeviceType=2
  in_STIMD.DM3_enable : KIBES_Signal/KIBES_Signal  MBDS_LibraryBlock=on  DatabaseKey=400  SignalName=STIMD.DM3_enable  SymbolName=STIMD_DM3_enable_000400  DataType=boolean  Init=0  Slope=1  Bias=0  DataSize=1  fpDataType=boolean  BlockIOType=Inport  DeviceType=2
  out_DCAN.GenericDM11RXMessage.DeviceEnable : KIBES_Signal/KIBES_Signal  MBDS_LibraryBlock=on  DatabaseKey=397  SignalName=DCAN.GenericDM11RXMessage.DeviceEnable  SymbolName=DCAN_GenericDM11RXMessage_DeviceEnable_000397  DataType=boolean  Init=0  Slope=1  Bias=0  DataSize=1  fpDataType=boolean  BlockIOType=Outport  DeviceType=0
  out_DCAN.GenericDM2TxMessage.Device_Enable : KIBES_Signal/KIBES_Signal  MBDS_LibraryBlock=on  DatabaseKey=393  SignalName=DCAN.GenericDM2TxMessage.Device_Enable  SymbolName=DCAN_GenericDM2TxMessage_Device_Enable_000393  DataType=boolean  Init=0  Slope=1  Bias=0  DataSize=1  fpDataType=boolean  BlockIOType=Outport  DeviceType=0
  out_DCAN.GenericDM3RxMessage.Device_Enable : KIBES_Signal/KIBES_Signal  MBDS_LibraryBlock=on  DatabaseKey=395  SignalName=DCAN.GenericDM3RxMessage.Device_Enable  SymbolName=DCAN_GenericDM3RxMessage_Device_Enable_000395  DataType=boolean  Init=0  Slope=1  Bias=0  DataSize=1  fpDataType=boolean  BlockIOType=Outport  DeviceType=0
  wires:
  Constant1/1 -> OR1/2(u2)
  OR1/1(y) -> out_DCAN.GenericDM11RXMessage.DeviceEnable/1
  in_STIMD.DM11_enable/1 -> OR1/1(u1)
  Constant2/1 -> OR2/2(u2)
  OR2/1(y) -> out_DCAN.GenericDM2TxMessage.Device_Enable/1
  in_STIMD.DM2_enable/1 -> OR2/1(u1)
  Constant3/1 -> OR3/2(u2)
  OR3/1(y) -> out_DCAN.GenericDM3RxMessage.Device_Enable/1
  in_STIMD.DM3_enable/1 -> OR3/1(u1)

== system APP_MyApplication/Model/APP_MyApplication_/DM4RX ==
  note: To Test with CAPL
      | F1 = 241  -- Normal Reply
      | F4 = 244  -- Short Reply Length
      | F5 = 245  --  ACK Negative (1)
      | F6 = 246  --  ACK Cannot Respond (3)
  note: App end
  note: TRUE   = SAE FORMAT
      | FALSE = MAN FORMAT
  Constant : Constant  InitFcn=|  Value=9  OutDataTypeStr=Inherit: Inherit via back propagation
      | if(exist('MBDS_BlockCallback', 'file'))
      |    MBDS_BlockCallback('Update', gcb);  
      | end
  Data Type Conversion : DataTypeConversion  InitFcn=|  SaturateOnIntegerOverflow=on
      | try
      |    MBDS_BlockCallback('Update', gcb);
      | end
      settings: AttributesFormatString=Saturate: %<SaturateOnIntegerOverflow>
  EQ : Subsystem  InitFcn=|  mask(EQ){MBDS_LibraryBlock=on, InputSameDT=on, MBDS_BlockVersion=08.20.02}
      | if(exist('MBDS_BlockCallback', 'file'))
      |    MBDS_BlockCallback('Update', gcb);
      | end
      mask prompts: MBDS_LibraryBlock "MBDS library block"; InputSameDT "Require all inputs to have the same data type"; MBDS_BlockVersion "Block version:"
      mask help: The block compares if both input signals are equal.
      mask init: same as APP_MyApplication/Model/APP_MyApplication_/OR
      mask Help: eval(['open([workdir(''library_dir:''),''\Blockset\help\'',get_param(gcb,''MaskType''),''.html''])'])
      mask Callback InputSameDT:
      | % Adopt value
      | if(exist('MBDS_BlockCallback', 'file'))
      |    MBDS_BlockCallback('InputSameDT', gcb);
      | end
      mask DialogControl ParameterTabVar0 Prompt: Signal Attributes
      mask DialogControl ParameterTabVar01 Prompt: Version
      mask Display:
      | % Show icon or block text
      | if(exist('MBDS_BlockCallback', 'file'))
      |    image(imread('EQ.tif','tif'),[0.35,0.35,0.355,0.25])
      |    disp('')
      | else
      |    disp(sprintf('=='));
      | end
  SRFlipFlop : Subsystem  InitFcn=|  mask(SRFlipFlop){MBDS_LibraryBlock=on, Q_Enabled=on, Not_Q_Enabled=off, MBDS_BlockVersion=08.20.02}
      | if(exist('MBDS_BlockCallback', 'file'))
      |    MBDS_BlockCallback('Update', gcb);
      | end
      mask prompts: MBDS_LibraryBlock "MBDS library block"; Q_Enabled "Show Q port"; Not_Q_Enabled "Show ~Q port"; MBDS_BlockVersion "Block version:"
      mask help: A flip flop. The set input (SET) dominates the reset input (RST).
      mask init: same as APP_MyApplication/Model/APP_MyApplication_/OR
      mask Help: eval(['open([workdir(''library_dir:''),''\Blockset\help\'',get_param(gcb,''MaskType''),''.html''])'])
      mask Callback Q_Enabled:
      | % Update mask parameter dialog
      | if(exist('MBDS_BlockCallback', 'file'))
      |    MBDS_BlockCallback('Q_Enabled', gcb);
      | end
      mask Callback Not_Q_Enabled:
      | % Update mask parameter dialog
      | if(exist('MBDS_BlockCallback', 'file'))
      |    MBDS_BlockCallback('Not_Q_Enabled', gcb);
      | end
      mask DialogControl ParameterTabVar0 Prompt: Main
      mask DialogControl ParameterTabVar01 Prompt: Version
      mask Display:
      | % Show icon or block text
      | if(exist('SRFlipFlop.tif', 'file'))
      |    image('SRFlipFlop.tif', [0.295739348370927 0.17 0.378947368421053 0.66]);
      |    disp('')
      | else
      |    disp(sprintf('SR\nFlipFlop'));
      | end
      | 
      | % Display port labels
      | port_label('input', 1, 'SET');
      | port_label('input', 2, 'RST');
      | port_label('output', 1, 'Q');
  in_DM4RXMainDevice.FaultIndication : KIBES_Signal/KIBES_Signal  MBDS_LibraryBlock=on  DatabaseKey=322  SignalName=DM4RXMainDevice.FaultIndication  SymbolName=DM4RXMainDevice_FaultIndication_000322  DataType=boolean  Init=0  Slope=1  Bias=0  DataSize=1  fpDataType=boolean  BlockIOType=Inport  DeviceType=0
  in_DM4RXMainDevice.FirstEntry : KIBES_Signal/KIBES_Signal  MBDS_LibraryBlock=on  DatabaseKey=323  SignalName=DM4RXMainDevice.FirstEntry  SymbolName=DM4RXMainDevice_FirstEntry_000323  DataType=boolean  Init=0  Slope=1  Bias=0  DataSize=1  fpDataType=boolean  BlockIOType=Inport  DeviceType=0
  in_DM4RXMainDevice.Fmi : KIBES_Signal/KIBES_Signal  MBDS_LibraryBlock=on  DatabaseKey=324  SignalName=DM4RXMainDevice.Fmi  SymbolName=DM4RXMainDevice_Fmi_000324  DataType=uint8  Init=0  Slope=1  Bias=0  DataSize=1  fpDataType=uint8  BlockIOType=Inport  DeviceType=0
  in_DM4RXMainDevice.LastEntry : KIBES_Signal/KIBES_Signal  MBDS_LibraryBlock=on  DatabaseKey=325  SignalName=DM4RXMainDevice.LastEntry  SymbolName=DM4RXMainDevice_LastEntry_000325  DataType=boolean  Init=0  Slope=1  Bias=0  DataSize=1  fpDataType=boolean  BlockIOType=Inport  DeviceType=0
  in_DM4RXMainDevice.NumberOfDtcs : KIBES_Signal/KIBES_Signal  MBDS_LibraryBlock=on  DatabaseKey=327  SignalName=DM4RXMainDevice.NumberOfDtcs  SymbolName=DM4RXMainDevice_NumberOfDtcs_000327  DataType=uint8  Init=0  Slope=1  Bias=0  DataSize=1  fpDataType=uint8  BlockIOType=Inport  DeviceType=0
  in_DM4RXMainDevice.OccCount : KIBES_Signal/KIBES_Signal  MBDS_LibraryBlock=on  DatabaseKey=328  SignalName=DM4RXMainDevice.OccCount  SymbolName=DM4RXMainDevice_OccCount_000328  DataType=uint8  Init=0  Slope=1  Bias=0  DataSize=1  fpDataType=uint8  BlockIOType=Inport  DeviceType=0
  in_DM4RXMainDevice.Spn : KIBES_Signal/KIBES_Signal  MBDS_LibraryBlock=on  DatabaseKey=331  SignalName=DM4RXMainDevice.Spn  SymbolName=DM4RXMainDevice_Spn_000331  DataType=uint32  Init=0  Slope=1  Bias=0  DataSize=1  fpDataType=uint32  BlockIOType=Inport  DeviceType=0
  in_PCAN.BusOffState : KIBES_Signal/KIBES_Signal  MBDS_LibraryBlock=on  DatabaseKey=638  SignalName=PCAN.BusOffState  SymbolName=PCAN_BusOffState_000638  DataType=boolean  Init=0  Slope=1  Bias=0  DataSize=1  fpDataType=boolean  BlockIOType=Inport  DeviceType=0
  in_PCAN.GenericDM4REQ.DeviceState : KIBES_Signal/KIBES_Signal  MBDS_LibraryBlock=on  DatabaseKey=319  SignalName=PCAN.GenericDM4REQ.DeviceState  SymbolName=PCAN_GenericDM4REQ_DeviceState_000319  DataType=uint16  Init=0  Slope=1  Bias=0  DataSize=1  fpDataType=uint16  BlockIOType=Inport  DeviceType=0
  in_STIMD.DM4RX_Device_Enable : KIBES_Signal/KIBES_Signal  MBDS_LibraryBlock=on  DatabaseKey=646  SignalName=STIMD.DM4RX_Device_Enable  SymbolName=STIMD_DM4RX_Device_Enable_000646  DataType=boolean  Init=0  Slope=1  Bias=0  DataSize=1  fpDataType=boolean  BlockIOType=Inport  DeviceType=2
  in_STIMD.DM4RX_EcuAddress : KIBES_Signal/KIBES_Signal  MBDS_LibraryBlock=on  DatabaseKey=333  SignalName=STIMD.DM4RX_EcuAddress  SymbolName=STIMD_DM4RX_EcuAddress_000333  DataType=uint8  Init=241  Slope=1  Bias=0  DataSize=1  fpDataType=uint8  BlockIOType=Inport  DeviceType=2
  in_STIMD.DM4RX_Next : KIBES_Signal/KIBES_Signal  MBDS_LibraryBlock=on  DatabaseKey=334  SignalName=STIMD.DM4RX_Next  SymbolName=STIMD_DM4RX_Next_000334  DataType=boolean  Init=0  Slope=1  Bias=0  DataSize=1  fpDataType=boolean  BlockIOType=Inport  DeviceType=2
  in_STIMD.DM4RX_Previous : KIBES_Signal/KIBES_Signal  MBDS_LibraryBlock=on  DatabaseKey=332  SignalName=STIMD.DM4RX_Previous  SymbolName=STIMD_DM4RX_Previous_000332  DataType=boolean  Init=0  Slope=1  Bias=0  DataSize=1  fpDataType=boolean  BlockIOType=Inport  DeviceType=2
  in_STIMD.DM4RX_RequestDm4 : KIBES_Signal/KIBES_Signal  MBDS_LibraryBlock=on  DatabaseKey=335  SignalName=STIMD.DM4RX_RequestDm4  SymbolName=STIMD_DM4RX_RequestDm4_000335  DataType=boolean  Init=0  Slope=1  Bias=0  DataSize=1  fpDataType=boolean  BlockIOType=Inport  DeviceType=2
  in_STIMD.DM4RX_SaeFormat : KIBES_Signal/KIBES_Signal  MBDS_LibraryBlock=on  DatabaseKey=442  SignalName=STIMD.DM4RX_SaeFormat  SymbolName=STIMD_DM4RX_SaeFormat_000442  DataType=boolean  Init=1  Slope=1  Bias=0  DataSize=1  fpDataType=boolean  BlockIOType=Inport  DeviceType=2
  out_DCAN.TX_Gen.DGenTx_5.MessageEnable : KIBES_Signal/KIBES_Signal  MBDS_LibraryBlock=on  DatabaseKey=643  SignalName=DCAN.TX_Gen.DGenTx_5.MessageEnable  SymbolName=DCAN_TX_Gen_DGenTx_5_MessageEnable_000643  DataType=boolean  Init=0  Slope=1  Bias=0  DataSize=1  fpDataType=boolean  BlockIOType=Outport  DeviceType=0
  out_DCAN.TX_Gen.DGenTx_5.ui_Val_02 : KIBES_Signal/KIBES_Signal  MBDS_LibraryBlock=on  DatabaseKey=645  SignalName=DCAN.TX_Gen.DGenTx_5.ui_Val_02  SymbolName=DCAN_TX_Gen_DGenTx_5_ui_Val_02_000645  DataType=uint16  Init=0  Slope=1  Bias=0  DataSize=1  fpDataType=uint16  BlockIOType=Outport  DeviceType=0
  out_DCAN.TX_Gen.DGenTx_5.usi_Val_01 : KIBES_Signal/KIBES_Signal  MBDS_LibraryBlock=on  DatabaseKey=644  SignalName=DCAN.TX_Gen.DGenTx_5.usi_Val_01  SymbolName=DCAN_TX_Gen_DGenTx_5_usi_Val_01_000644  DataType=uint8  Init=0  Slope=1  Bias=0  DataSize=1  fpDataType=uint8  BlockIOType=Outport  DeviceType=0
  out_DM4RXMainDevice.EcuAddress : KIBES_Signal/KIBES_Signal  MBDS_LibraryBlock=on  DatabaseKey=321  SignalName=DM4RXMainDevice.EcuAddress  SymbolName=DM4RXMainDevice_EcuAddress_000321  DataType=uint8  Init=0  Slope=1  Bias=0  DataSize=1  fpDataType=uint8  BlockIOType=Outport  DeviceType=0
  out_DM4RXMainDevice.NextEntry : KIBES_Signal/KIBES_Signal  MBDS_LibraryBlock=on  DatabaseKey=326  SignalName=DM4RXMainDevice.NextEntry  SymbolName=DM4RXMainDevice_NextEntry_000326  DataType=boolean  Init=0  Slope=1  Bias=0  DataSize=1  fpDataType=boolean  BlockIOType=Outport  DeviceType=0
  out_DM4RXMainDevice.PreviousEntry : KIBES_Signal/KIBES_Signal  MBDS_LibraryBlock=on  DatabaseKey=329  SignalName=DM4RXMainDevice.PreviousEntry  SymbolName=DM4RXMainDevice_PreviousEntry_000329  DataType=boolean  Init=0  Slope=1  Bias=0  DataSize=1  fpDataType=boolean  BlockIOType=Outport  DeviceType=0
  out_DM4RXMainDevice.SAEJ1939Format : KIBES_Signal/KIBES_Signal  MBDS_LibraryBlock=on  DatabaseKey=330  SignalName=DM4RXMainDevice.SAEJ1939Format  SymbolName=DM4RXMainDevice_SAEJ1939Format_000330  DataType=boolean  Init=0  Slope=1  Bias=0  DataSize=1  fpDataType=boolean  BlockIOType=Outport  DeviceType=0
  out_PCAN.GenericDM4REQ.DeviceEnable : KIBES_Signal/KIBES_Signal  MBDS_LibraryBlock=on  DatabaseKey=318  SignalName=PCAN.GenericDM4REQ.DeviceEnable  SymbolName=PCAN_GenericDM4REQ_DeviceEnable_000318  DataType=boolean  Init=0  Slope=1  Bias=0  DataSize=1  fpDataType=boolean  BlockIOType=Outport  DeviceType=0
  out_PCAN.GenericDM4REQ.RequestDM4 : KIBES_Signal/KIBES_Signal  MBDS_LibraryBlock=on  DatabaseKey=320  SignalName=PCAN.GenericDM4REQ.RequestDM4  SymbolName=PCAN_GenericDM4REQ_RequestDM4_000320  DataType=boolean  Init=0  Slope=1  Bias=0  DataSize=1  fpDataType=boolean  BlockIOType=Outport  DeviceType=0
  out_RAMDevice.DM4RX_BusOff_GeneralError : KIBES_Signal/KIBES_Signal  MBDS_LibraryBlock=on  DatabaseKey=647  SignalName=RAMDevice.DM4RX_BusOff_GeneralError  SymbolName=RAMDevice_DM4RX_BusOff_GeneralError_000647  DataType=boolean  Init=0  Slope=1  Bias=0  DataSize=1  fpDataType=boolean  BlockIOType=Outport  DeviceType=0
  wires:
  in_STIMD.DM4RX_SaeFormat/1 -> out_DM4RXMainDevice.SAEJ1939Format/1
  in_STIMD.DM4RX_Next/1 -> out_DM4RXMainDevice.NextEntry/1
  in_STIMD.DM4RX_Previous/1 -> out_DM4RXMainDevice.PreviousEntry/1
  in_STIMD.DM4RX_EcuAddress/1 -> out_DM4RXMainDevice.EcuAddress/1
  in_STIMD.DM4RX_RequestDm4/1 -> SRFlipFlop/2(RST), out_PCAN.GenericDM4REQ.RequestDM4/1
  in_STIMD.DM4RX_Device_Enable/1 -> out_DCAN.TX_Gen.DGenTx_5.MessageEnable/1, out_PCAN.GenericDM4REQ.DeviceEnable/1
  in_PCAN.GenericDM4REQ.DeviceState/1 -> EQ/1(u1), out_DCAN.TX_Gen.DGenTx_5.ui_Val_02/1
  Data Type Conversion/1 -> out_DCAN.TX_Gen.DGenTx_5.usi_Val_01/1
  in_PCAN.BusOffState/1 -> Data Type Conversion/1
  EQ/1(y) -> SRFlipFlop/1(SET)
  Constant/1 -> EQ/2(u2)
  SRFlipFlop/1(Q) -> out_RAMDevice.DM4RX_BusOff_GeneralError/1

== system APP_MyApplication/Model/APP_MyApplication_/DR-CAN(6) ==
  note: 18010621
  Constant1 : Constant  InitFcn=|  Value=66  OutDataTypeStr=uint8
      | if(exist('MBDS_BlockCallback', 'file'))
      |    MBDS_BlockCallback('Update', gcb);  
      | end
  Constant3 : Constant  InitFcn=|  OutDataTypeStr=boolean
      | if(exist('MBDS_BlockCallback', 'file'))
      |    MBDS_BlockCallback('Update', gcb);  
      | end
  in_DRCAN.TX_GEN.DRGenTX_1.MessageState : KIBES_Signal/KIBES_Signal  MBDS_LibraryBlock=on  DatabaseKey=301  SignalName=DRCAN.TX_GEN.DRGenTX_1.MessageState  SymbolName=DRCAN_TX_GEN_DRGenTX_1_MessageState_000301  DataType=uint16  Init=0  Slope=1  Bias=0  DataSize=1  fpDataType=uint16  BlockIOType=Inport  DeviceType=0
  out_DRCAN.TX_GEN.DRGenTX_1.MessageEnable : KIBES_Signal/KIBES_Signal  MBDS_LibraryBlock=on  DatabaseKey=300  SignalName=DRCAN.TX_GEN.DRGenTX_1.MessageEnable  SymbolName=DRCAN_TX_GEN_DRGenTX_1_MessageEnable_000300  DataType=boolean  Init=0  Slope=1  Bias=0  DataSize=1  fpDataType=boolean  BlockIOType=Outport  DeviceType=0
  out_DRCAN.TX_GEN.DRGenTX_1.Val_1 : KIBES_Signal/KIBES_Signal  MBDS_LibraryBlock=on  DatabaseKey=302  SignalName=DRCAN.TX_GEN.DRGenTX_1.Val_1  SymbolName=DRCAN_TX_GEN_DRGenTX_1_Val_1_000302  DataType=uint8  Init=0  Slope=1  Bias=0  DataSize=1  fpDataType=uint8  BlockIOType=Outport  DeviceType=0
  wires:
  Constant3/1 -> out_DRCAN.TX_GEN.DRGenTX_1.MessageEnable/1
  Constant1/1 -> out_DRCAN.TX_GEN.DRGenTX_1.Val_1/1
